simulink model "LocomotionSubsystem_StateFeedBackControl"  (R2019b)
settings: Solver=VariableStepAuto  StartTime=0.0  StopTime=42  RelTol=1e-3
libraries: mobileRoboticsLib x4, simulink x2, robotalgslib x1
settings Model: Creator=Nathanael  LastModifiedBy=Nathanael

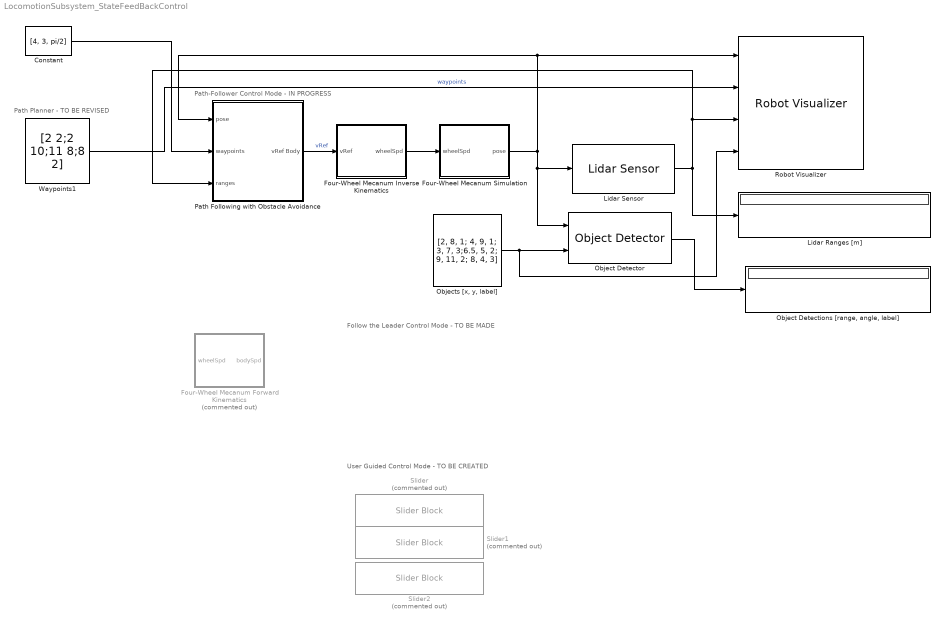
== system LocomotionSubsystem_StateFeedBackControl ==
  note: Path Planner - TO BE REVISED
  note: Path-Follower Control Mode - IN PROGRESS
  note: Follow the Leader Control Mode - TO BE MADE
  note: User Guided Control Mode - TO BE CREATED
  Constant : Constant  Value=[4, 3, pi/2]
  Four-Wheel Mecanum Forward Kinematics : Subsystem  Commented=on  AncestorBlock=mobileRoboticsLib/Kinematic Models/Four-Wheel Mecanum/Four-Wheel Mecanum Forward Kinematics  mask(Four-Wheel Mecanum Forward Kinematics){wheelRadius=0.1, wheelBase=0.4, wheelTrack=0.5}
      mask prompts: wheelRadius "Wheel Radius [m]"; wheelBase "Wheelbase [m]"; wheelTrack "Track [m]"
      mask help:
      | Calculates the forward kinematics for a four-wheeled vehicle with Mecanum wheels.
      |
      | Input: Wheel speeds [w1; w2; w3; w4] (rad/s)
      |
      | Output: Vehicle velocities [vx; vy; w] in body coordinates (m/s, m/s, and rad/s)
      mask Help: web('matlab:edit mrsDocFourWheelMecanum')
  Four-Wheel Mecanum Inverse Kinematics : Subsystem  AncestorBlock=mobileRoboticsLib/Kinematic Models/Four-Wheel Mecanum/Four-Wheel Mecanum Inverse Kinematics  mask(Four-Wheel Mecanum Inverse Kinematics){wheelRadius=0.1, wheelBase=0.535, wheelTrack=0.459}
      mask prompts: wheelRadius "Wheel Radius [m]"; wheelBase "Wheelbase [m]"; wheelTrack "Track [m]"
      mask help:
      | Calculates the inverse kinematics for a four-wheeled vehicle with Mecanum wheels.
      |
      | Input: Vehicle velocities [vx; vy; w] in body coordinates (m/s, m/s, and rad/s)
      |
      | Output: Wheel speeds [w1; w2; w3; w4] (rad/s)
      mask Help: web('matlab:edit mrsDocFourWheelMecanum')
  Four-Wheel Mecanum Simulation : Subsystem  AncestorBlock=mobileRoboticsLib/Kinematic Models/Four-Wheel Mecanum/Four-Wheel Mecanum Simulation  mask(Four-Wheel Mecanum Simulation){wheelRadius=0.1, wheelBase=0.535, wheelTrack=0.459, initX=1, initY=1, initAngle=0, Ts=0.05}
      mask prompts: wheelRadius "Wheel Radius [m]"; wheelBase "Wheelbase [m]"; wheelTrack "Track [m]"; initX "Initial X Position [m]"; initY "Initial Y Position [m]"; initAngle "Initial Angle [rad]"; Ts "Sample Time"
      mask help:
      | Simulates the kinematics of a four-wheeled vehicle with Mecanum wheels, from a specified initial pose.
      |
      | Input: Wheel speeds [w1; w2; w3; w4] (rad/s)
      |
      | Output: Pose [x; y; theta], in m, m, and rad
      |
      | Set the Sample Time parameter to 0 for continuous-time simulation, or a positive number for discrete-time simulation.
      mask Help: web('matlab:edit mrsDocFourWheelMecanum')
      mask Callback Ts:
      | Ts = evalin('base',get_param(gcb,'Ts'));
      | blk = [gcb '/Generic Robot Simulation/Velocity Integrator'];
      | if Ts > 0
      |     set_param(blk,'OverrideUsingVariant','mode==2');
      | else
      |     set_param(blk,'OverrideUsingVariant','mode==1');
      | end
  Lidar Ranges [m] : Display
  Lidar Sensor : mobileRoboticsLib/Environments/Lidar Sensor  mapName=test_map  sensorOffset=[ 0, 0 ]  scanAngles=[ -pi/4, 0, pi/4 ]  maxRange=5
      settings: SourceProductName=Mobile Robotics Simulation Toolbox
  "Object Detections [range, angle, label]" : Display
  Object Detector : mobileRoboticsLib/Environments/Object Detector  mapName=test_map  sensorOffset=[ 0, 0 ]  sensorAngle=0  fieldOfView=pi/3  maxRange=5  maxDetections=3  sampleTime=0.1
      settings: SourceProductName=Mobile Robotics Simulation Toolbox
  "Objects [x, y, label]" : Constant  Value=[2, 8, 1; 4, 9, 1; 3, 7, 3;6.5, 5, 2; 9, 11, 2; 8, 4, 3]
  Path Following with Obstacle Avoidance : Subsystem
  Robot Visualizer : mobileRoboticsLib/Environments/Robot Visualizer  robotRadius=0.5  mapName=map  showTrajectory=on  hasWaypoints=on  hasLidar=on  sensorOffset=[ 0, 0 ]  scanAngles=[ -pi/4, 0, pi/4 ]  hasObjDetector=on  objDetectorOffset=[ 0, 0 ]  objDetectorAngle=0  objDetectorFOV=pi/4  objDetectorMaxRange=5  objectColors=[ 1, 0, 0; 0, 1, 0; 0, 0, 1 ]  objectMarkers=s
  Slider : SliderBlock  Commented=on
  Slider1 : SliderBlock  Commented=on
  Slider2 : SliderBlock  Commented=on
  Waypoints1 : Constant  Value=[2 2;2 10;11 8;8 2]
  wires:
  Four-Wheel Mecanum Simulation/1(pose) -> Path Following with Obstacle Avoidance/1(pose), Robot Visualizer/1, Object Detector/1, Lidar Sensor/1
  Four-Wheel Mecanum Inverse Kinematics/1(wheelSpd) -> Four-Wheel Mecanum Simulation/1(wheelSpd)
  Path Following with Obstacle Avoidance/1(vRef Body) -> Four-Wheel Mecanum Inverse Kinematics/1(vRef)  "vRef"
  Waypoints1/1 -> Robot Visualizer/2  "waypoints"
  Lidar Sensor/1 -> Path Following with Obstacle Avoidance/3(ranges), Robot Visualizer/3, Lidar Ranges [m]/1
  "Objects [x, y, label]"/1 -> Robot Visualizer/4, Object Detector/2
  Object Detector/1 -> "Object Detections [range, angle, label]"/1
  Constant/1 -> Path Following with Obstacle Avoidance/2(waypoints)

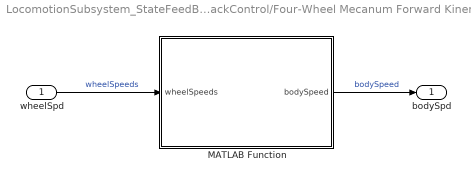
== system LocomotionSubsystem_StateFeedBackControl/Four-Wheel Mecanum Forward Kinematics ==
  wheelSpd : Inport
  MATLAB Function : MATLAB Function  TreatAsAtomicUnit=on
  bodySpd : Outport  VectorParamsAs1DForOutWhenUnconnected=off
  wires:
  wheelSpd/1 -> MATLAB Function/1(wheelSpeeds)  "wheelSpeeds"
  MATLAB Function/1(bodySpeed) -> bodySpd/1  "bodySpeed"

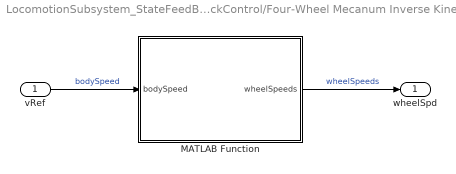
== system LocomotionSubsystem_StateFeedBackControl/Four-Wheel Mecanum Inverse Kinematics ==
  vRef : Inport
  MATLAB Function : MATLAB Function  TreatAsAtomicUnit=on
  wheelSpd : Outport  VectorParamsAs1DForOutWhenUnconnected=off
  wires:
  MATLAB Function/1(wheelSpeeds) -> wheelSpd/1  "wheelSpeeds"
  vRef/1 -> MATLAB Function/1(bodySpeed)  "bodySpeed"

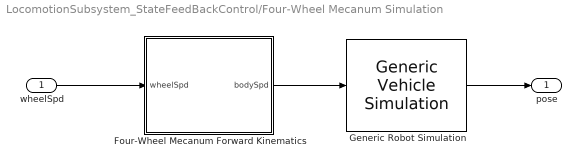
== system LocomotionSubsystem_StateFeedBackControl/Four-Wheel Mecanum Simulation ==
  wheelSpd : Inport
  Four-Wheel Mecanum Forward Kinematics : Subsystem  AncestorBlock=mobileRoboticsLib/Kinematic Models/Four-Wheel Mecanum/Four-Wheel Mecanum Forward Kinematics  mask(Four-Wheel Mecanum Forward Kinematics){wheelRadius=0.1, wheelBase=0.535, wheelTrack=0.459}
      mask prompts: wheelRadius "Wheel Radius [m]"; wheelBase "Wheelbase [m]"; wheelTrack "Track [m]"
      mask help:
      | Calculates the forward kinematics for a four-wheeled vehicle with Mecanum wheels.
      |
      | Input: Wheel speeds [w1; w2; w3; w4] (rad/s)
      |
      | Output: Vehicle velocities [vx; vy; w] in body coordinates (m/s, m/s, and rad/s)
      mask Help: web('matlab:edit mrsDocFourWheelMecanum')
  Generic Robot Simulation : mobileRoboticsLib/Utilities/Generic Vehicle Simulation  initX=initX  initY=initY  initAngle=initAngle  Ts=Ts
      link override Velocity Integrator: LabelModeActiveChoice=mode==2
      settings: SourceProductName=Mobile Robotics Simulation Toolbox
  pose : Outport  VectorParamsAs1DForOutWhenUnconnected=off
  wires:
  wheelSpd/1 -> Four-Wheel Mecanum Forward Kinematics/1(wheelSpd)
  Four-Wheel Mecanum Forward Kinematics/1(bodySpd) -> Generic Robot Simulation/1
  Generic Robot Simulation/1 -> pose/1

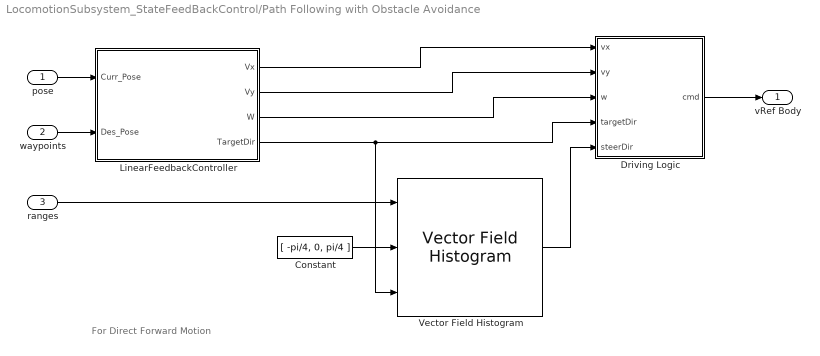
== system LocomotionSubsystem_StateFeedBackControl/Path Following with Obstacle Avoidance ==
  note: For Direct Forward Motion
  pose : Inport
  waypoints : Inport  Port=2
  ranges : Inport  Port=3
  Constant : Constant  Value=[ -pi/4, 0, pi/4 ]
  Driving Logic : Subsystem
  LinearFeedbackController : MATLAB Function  TreatAsAtomicUnit=on
  Vector Field Histogram : robotalgslib/Vector Field Histogram  NumAngularSectors=36  DistanceLimits=[ 0.05, 3 ]  HistogramThresholds=[ 5, 10 ]  RobotRadius=0.5  SafetyDistance=0.6  MinTurningRadius=0  SimulateUsing=Interpreted execution  TargetDirectionWeight=5  CurrentDirectionWeight=2  PreviousDirectionWeight=2
      settings: SourceProductName=Robotics System Toolbox  SourceProductBaseCode=RO
  vRef Body : Outport  VectorParamsAs1DForOutWhenUnconnected=off
  wires:
  Driving Logic/1(cmd) -> vRef Body/1
  waypoints/1 -> LinearFeedbackController/2(Des_Pose)
  ranges/1 -> Vector Field Histogram/1
  Vector Field Histogram/1 -> Driving Logic/5(steerDir)
  Constant/1 -> Vector Field Histogram/2
  LinearFeedbackController/1(Vx) -> Driving Logic/1(vx)
  LinearFeedbackController/4(TargetDir) -> Driving Logic/4(targetDir), Vector Field Histogram/3
  pose/1 -> LinearFeedbackController/1(Curr_Pose)
  LinearFeedbackController/2(Vy) -> Driving Logic/2(vy)
  LinearFeedbackController/3(W) -> Driving Logic/3(w)

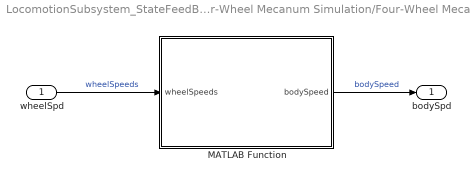
== system LocomotionSubsystem_StateFeedBackControl/Four-Wheel Mecanum Simulation/Four-Wheel Mecanum Forward Kinematics ==
  wheelSpd : Inport
  MATLAB Function : MATLAB Function  TreatAsAtomicUnit=on
  bodySpd : Outport  VectorParamsAs1DForOutWhenUnconnected=off
  wires:
  MATLAB Function/1(bodySpeed) -> bodySpd/1  "bodySpeed"
  wheelSpd/1 -> MATLAB Function/1(wheelSpeeds)  "wheelSpeeds"

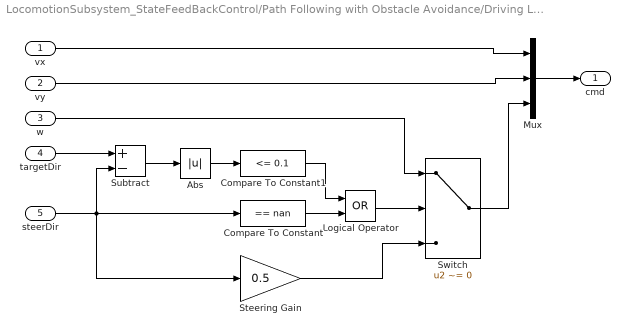
== system LocomotionSubsystem_StateFeedBackControl/Path Following with Obstacle Avoidance/Driving Logic ==
  vx : Inport
  vy : Inport  Port=2
  w : Inport  Port=3
  targetDir : Inport  Port=4
  steerDir : Inport  Port=5
  Abs : Abs
  Compare To Constant : simulink/Logic and Bit Operations/Compare To Constant  relop===  const=nan  OutDataTypeStr=boolean
  Compare To Constant1 : simulink/Logic and Bit Operations/Compare To Constant  relop=<=  const=0.1  OutDataTypeStr=boolean
  Logical Operator : Logic  Operator=OR  AllPortsSameDT=off  OutDataTypeStr=boolean
  Mux : Mux  Inputs=3
  Steering Gain : Gain  Gain=0.5
  Subtract : Sum  Inputs=+-
  Switch : Switch  Criteria=u2 ~= 0
  cmd : Outport  VectorParamsAs1DForOutWhenUnconnected=off
  wires:
  Steering Gain/1 -> Switch/3
  w/1 -> Switch/1
  Logical Operator/1 -> Switch/2
  Mux/1 -> cmd/1
  Compare To Constant1/1 -> Logical Operator/1
  Abs/1 -> Compare To Constant1/1
  Subtract/1 -> Abs/1
  targetDir/1 -> Subtract/1
  Compare To Constant/1 -> Logical Operator/2
  steerDir/1 -> Compare To Constant/1, Subtract/2, Steering Gain/1
  vx/1 -> Mux/1
  Switch/1 -> Mux/3
  vy/1 -> Mux/2

== matlab function LocomotionSubsystem_StateFeedBackControl/Four-Wheel Mecanum Forward Kinematics/MATLAB Function ==
  settings: updateMethod=DISCRETE
  data: wheelSpeeds input; bodySpeed output; wheelRadius parameter; wheelBase parameter; wheelTrack parameter
function bodySpeed = fourWheelMecanumFwdKin(wheelSpeeds,wheelRadius,wheelBase,wheelTrack)
    
    % Initialize FourWheelMecanum object
    persistent robot
    if isempty(robot)
        robot = FourWheelMecanum_toolbox(wheelRadius,wheelBase,wheelTrack);
    end
    
    % Run object's forward kinematics method
    bodySpeed = forwardKinematics(robot,wheelSpeeds);

end

== matlab function LocomotionSubsystem_StateFeedBackControl/Path Following with Obstacle Avoidance/LinearFeedbackController ==
  data: Curr_Pose input; Vx output; Des_Pose input; Vy output; W output; TargetDir output
function [Vx, Vy, W, TargetDir] = LinearFeedbackController(Curr_Pose, Des_Pose)
%LINEARFEEDBACKCONTROL - Linearization Feedback Control for Omnidirectional
%Robot (Ex. 4 Wheeled Mecanum Robot)
%   Inputs: Current Pose, Desired Path
%   Outputs: Control Body Velocity

%Des_Pose = transpose(Des_Pose);
TargetDir =atan((Curr_Pose(2) - Des_Pose(2))/(Curr_Pose(1) - Des_Pose(1)));
A = [10, 0, 0; 0, 10, 0; 0, 0, 0.5]; % A(Curr_Pose - Des_Pose)
%A = [-3.327, 1.147, 1.154; 1.147, -1.078, -1.329; 1.154, -1.329, -3.048]; % A(Curr_Pose - Des_Pose)
%A = [3, 6, 0; 3, 9, 0; 0, 3, 6]; % A(Curr_Pose - Des_Pose)
err = (Des_Pose - Curr_Pose);
if norm(err(1:2)) < 0.01
    err(1) = 0;
    err(2) = 0;
end
Vel = A*err;
if norm(Vel(1:2)) > 1.5
    Unit = [Vel(1)/norm(Vel(1:2)),Vel(2)/norm(Vel(1:2))];
    Vx = Unit(1)*1.5;
    Vy = Unit(2)*1.5;
else
    Vx = Vel(1);
    Vy = Vel(2);
end

W = Vel(3);
if W > 0.2
    W = 0.2; % Max Ang Vel
end

end

== matlab function LocomotionSubsystem_StateFeedBackControl/Four-Wheel Mecanum Simulation/Four-Wheel Mecanum Forward Kinematics/MATLAB Function ==
  settings: updateMethod=DISCRETE
  data: wheelSpeeds input; bodySpeed output; wheelRadius parameter; wheelBase parameter; wheelTrack parameter
function bodySpeed = fourWheelMecanumFwdKin(wheelSpeeds,wheelRadius,wheelBase,wheelTrack)
    
    % Initialize FourWheelMecanum object
    persistent robot
    if isempty(robot)
        robot = FourWheelMecanum_toolbox(wheelRadius,wheelBase,wheelTrack);
    end
    
    % Run object's forward kinematics method
    bodySpeed = forwardKinematics(robot,wheelSpeeds);

end

== matlab function LocomotionSubsystem_StateFeedBackControl/Four-Wheel Mecanum Inverse Kinematics/MATLAB Function ==
  data: bodySpeed input; wheelRadius parameter; wheelSpeeds output; wheelBase parameter; wheelTrack parameter
function wheelSpeeds = fourWheelMecanumInvKin(bodySpeed,wheelRadius,wheelBase,wheelTrack)
    
    % Initialize FourWheelMecanum object
    persistent robot
    if isempty(robot)
        robot = FourWheelMecanum_toolbox(wheelRadius,wheelBase,wheelTrack);
    end
    
    % Run object's inverse kinematics method
    wheelSpeeds = inverseKinematics(robot,bodySpeed);

end
